simulink model "Path_Planning"  (R2014a)
settings: Solver=ode45  StartTime=0.0  StopTime=15  RelTol=1e-3
InitFcn:
  | run('head.m')
values from neighbouring files (symbols this model uses):
  d = 0.235    [head.m]
libraries: simulink x1
settings Model: Creator=WXY  LastModifiedBy=Tim

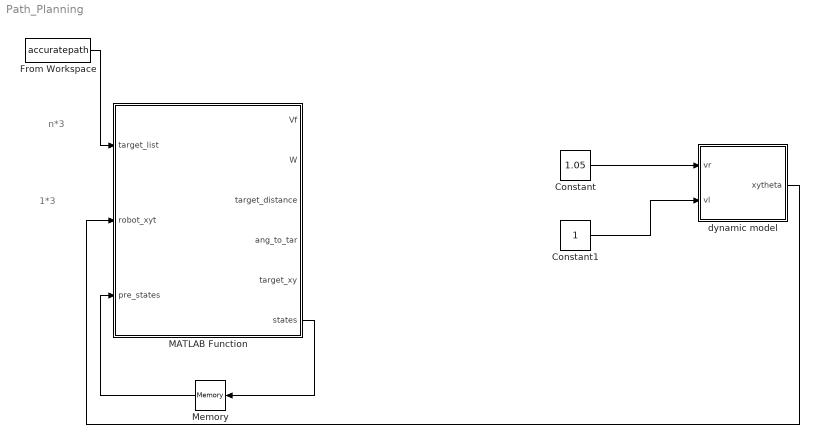
== system Path_Planning ==
  note: n*3
  note: 1*3
  Constant : Constant  Value=1.05
  Constant1 : Constant
  From Workspace : FromWorkspace  VariableName=accuratepath  SampleTime=0
  MATLAB Function : MATLAB Function  TreatAsAtomicUnit=on
  Memory : Memory  X0=[0]
  dynamic model : Subsystem
  wires:
  Constant/1 -> dynamic model/1(vr)
  Constant1/1 -> dynamic model/2(vl)
  MATLAB Function/6(states) -> Memory/1
  Memory/1 -> MATLAB Function/3(pre_states)
  dynamic model/1(xytheta) -> MATLAB Function/2(robot_xyt)
  From Workspace/1 -> MATLAB Function/1(target_list)

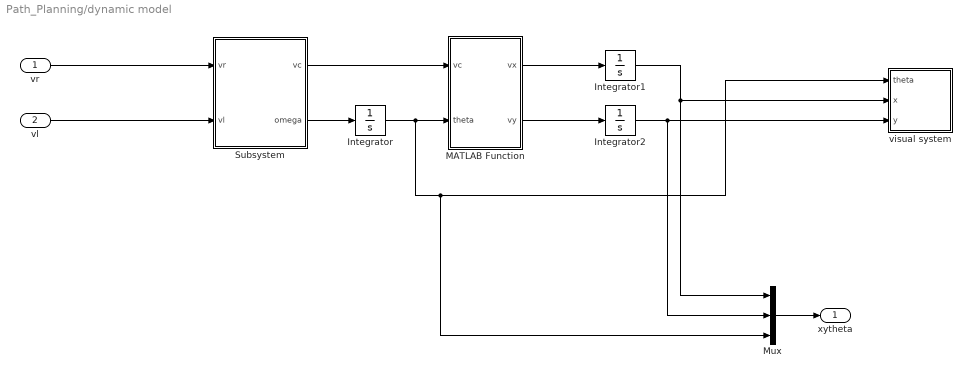
== system Path_Planning/dynamic model ==
  vr : Inport
  vl : Inport  Port=2
  Integrator : Integrator
  Integrator1 : Integrator
  Integrator2 : Integrator
  MATLAB Function : MATLAB Function  TreatAsAtomicUnit=on
  Mux : Mux  Inputs=3
  Subsystem : Subsystem
  visual system : Subsystem
  xytheta : Outport
  wires:
  MATLAB Function/2(vy) -> Integrator2/1
  MATLAB Function/1(vx) -> Integrator1/1
  vr/1 -> Subsystem/1(vr)
  vl/1 -> Subsystem/2(vl)
  Subsystem/1(vc) -> MATLAB Function/1(vc)
  Subsystem/2(omega) -> Integrator/1
  Mux/1 -> xytheta/1
  Integrator/1 -> Mux/3, visual system/1(theta), MATLAB Function/2(theta)
  Integrator1/1 -> visual system/2(x), Mux/1
  Integrator2/1 -> Mux/2, visual system/3(y)

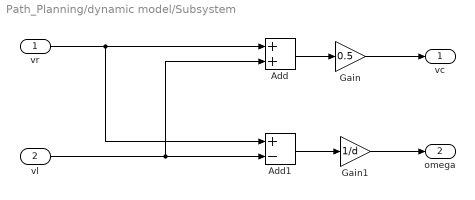
== system Path_Planning/dynamic model/Subsystem ==
  vr : Inport
  vl : Inport  Port=2
  Add : Sum
  Add1 : Sum  Inputs=+-
  Gain : Gain  Gain=0.5
  Gain1 : Gain  Gain=1/d
  vc : Outport
  omega : Outport  Port=2
  wires:
  vl/1 -> Add1/2, Add/2
  Gain/1 -> vc/1
  Add1/1 -> Gain1/1
  Add/1 -> Gain/1
  Gain1/1 -> omega/1
  vr/1 -> Add1/1, Add/1

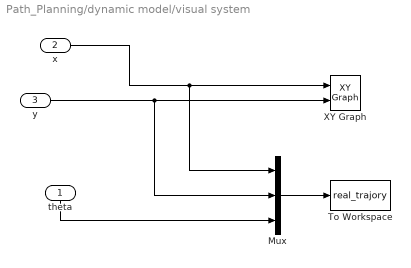
== system Path_Planning/dynamic model/visual system ==
  theta : Inport
  x : Inport  Port=2
  y : Inport  Port=3
  Mux : Mux  Inputs=3
  To Workspace : ToWorkspace  VariableName=real_trajory  SaveFormat=Structure With Time  SampleTime=-1
  XY Graph : simulink/Sinks/XY Graph  xmin=-10  xmax=10  ymin=-10  ymax=10  st=-1
  wires:
  Mux/1 -> To Workspace/1
  theta/1 -> Mux/3
  x/1 -> Mux/1, XY Graph/1
  y/1 -> Mux/2, XY Graph/2

== matlab function Path_Planning/MATLAB Function ==
  data: target_list input; Vf output; robot_xyt input; pre_states input; W output; target_distance output; ang_to_tar output; target_xy output; states output
function [Vf, W, target_distance, ang_to_tar, target_xy, states] = ...
    WaypointControl(target_list, robot_xyt, pre_states)
vlimit = 0.5; %最大限速
dist_thr = 0.1;
ang_thr = 10*pi/180;
method = 1;
step = 3; % 预估目标点的间隔
Kv_1 = 0.7; % 左轮速度常数   目标v=kv*x
Kw_1 = 0.45; % 左轮转角速度常数  目标w=kw*x
Kv_2 = 0.2;
Kw_2 = 0.9;
Psi_d = pi; % 机器人最终停止时角度（朝向）

% 初始化输出参数
 Vf=0;
 W=0;
 finished_path_flag=0; 
 
 persistent Vf_1 end_flag;
 
 if isempty(Vf_1)
     Vf_1=0;
 end
 if isempty(end_flag)
    end_flag = 0;
 end
states = pre_states;

rx = robot_xyt(1);
ry = robot_xyt(2);
rtheta = check_angle(robot_xyt(3));
target_xy = [rx ry];  %当前目标x y
[n xy] = size(target_list);
if n==2 && xy==1
    target_xy = [target_list(1,1) target_list(2,1)];
    n = 1;
else
    for i=1:n
        if states(1) == i
            for j=1:xy
                target_xy(j) = target_list(i, j);
            end
        end
    end
end

tx = target_xy(1);
ty = target_xy(2);
target_distance = find_dist(rx, ry, tx, ty);
ang_to_tar= find_theta(rx, ry, rtheta, tx, ty);

if ((states(1) == n) && (target_distance <= dist_thr))  %到达终点或离终点

        Vf=0;
        W=0;
        
       if (end_flag == 1) && (target_distance <= dist_thr) % 最终到达目的地时朝向转到要求位置
            [Vf, W] = ClosedLoop_Sequential(0, check_angle(check_angle(Psi_d)-check_angle(rtheta)), vlimit, ang_thr, dist_thr, Kv_1, Kw_1, Vf_1); 
             Vf_1=Vf;
       end
   
else
    % 找到目标点
    if (target_distance <= dist_thr) && (end_flag==0)
            states(1) = pre_states(1) + step;%1;
      if( pre_states(1) > 0 )      
         while (abs((target_list(states(1),1))-(target_list(pre_states(1),1)))<2*dist_thr) && (abs((target_list(states(1),2))-(target_list(pre_states(1),2)))<2*dist_thr)
             if (states(1)<=(n-step))
                 states(1) = states(1) + step;%1;
             else
                 states(1)=n;
             end
         end
      else
          states(1)=states(1)+step;
      end
         if states(1) >= n 
            states(1) = n;
            end_flag=1;
         end
        
    else
        if method == 2
            [Vf, W] = ClosedLoop_Both(target_distance,  ang_to_tar, vlimit, Kv_2, Kw_2);    
        else
            [Vf, W] = ClosedLoop_Sequential(target_distance,  ang_to_tar, vlimit, ang_thr, dist_thr, Kv_1, Kw_1, Vf_1); 
            Vf_1=Vf;
        end       
    end
end

return;

% 认为机器人转角应在-180到180度之间
function [y] = check_angle(x)
y = x;
while ( x > pi || x < -pi)
    if x > pi
        y = x - 2*pi;
    else
        y = x + 2*pi;
    end
end
return;

% 目标点与当前点距离
function dist = find_dist(rx, ry, tx, ty)
dist = sqrt((rx-tx)^2 + (ry-ty)^2);
return;

% 机器人当前需要转过的角度
function [theta]= find_theta(rx, ry, rtheta, tx, ty)

X = tx - rx;
Y = ty - ry;
theta = atan2(Y, X);
theta = check_angle(check_angle(theta)-check_angle(rtheta));

return;

% 根据目标距离和转角算出机器人的前进速度和转角速度
function [Vf, W] = ClosedLoop_Both(dist, theta, vlimit, Kv,Kw)

d = 0.23;
vmax = vlimit;
wmax = (2*vmax);
W = Kw*theta;

Vf = Kv * dist;

w_sign = sign(W); % 保留转角符号
if abs(W) > wmax
    W = w_sign*wmax;
end
if abs(Vf)> vlimit
    Vf = sign(Vf)*vlimit;%%%%% Vf = abs(Vf)*vlimit;
end

return;

% 仅前进或仅转弯
function [Vf, W] = ClosedLoop_Sequential(dist, theta, vlimit, ang_thr, dist_thr, Kv, Kw, Vf_1)

d = 0.23;
vmax = vlimit;
wmax = (2*vmax);

if (((abs(theta) > ang_thr))  && (Vf_1<0.01)) || (abs(theta) > 5*ang_thr) 
        W=Kw*theta;
        Vf=0;
        if abs(W)> wmax
            W=sign(W)*wmax;
        end
else
        Vf=Kv*dist;
       
        if abs(Vf)>vlimit
            Vf=sign(Vf)*vlimit;
        end
        
        W=0;
        
end

return;

== matlab function Path_Planning/dynamic model/MATLAB Function ==
  data: vc input; vx output; theta input; vy output
function [vx,vy] = fcn(vc,theta)
%#codegen

vx=vc*cos(theta);
vy=vc*sin(theta);

end
